simulink model "TempControl_ClosedLoop"  (R2025b)
settings: Solver=FixedStepAuto  StartTime=0.0  StopTime=1000  FixedStep=10e-3  RelTol=1e-3  EnableMultiTasking=on
libraries: mbedblockslib x2
settings Model: ExtModeTrigDuration=10  Creator=Lukas  LastModifiedBy=matte
settings OptimizationCC: EnhancedBackFolding=on  PassReuseOutputArgsAs=Individual arguments  ZeroExternalMemoryAtStartup=off  ZeroInternalMemoryAtStartup=off  MaxStackSize=64  OptimizeBlockOrder=speed  DifferentSizesBufferReuse=on  OptimizationCustomize=off  EfficientTunableParamExpr=on
settings DebuggingCC: ParameterTunabilityLossMsg=error
settings HardwareCC: ProdBitPerPointer=32.0  ProdBitPerSizeT=32.0  ProdBitPerPtrDiffT=32.0  ProdLargestAtomicInteger=Long  ProdLargestAtomicFloat=Double  ProdWordSize=32.0  ProdLongLongMode=on  ProdHWDeviceType=ARM Compatible->ARM Cortex
settings SFSimCC: MATLABDynamicMemAlloc=off
settings RTWCC: SystemTargetFile=ert.tlc  HardwareBoard=STM32 Nucleo F401RE  TemplateMakefile=ert_default_tmf  Toolchain=GNU Tools for ARM Embedded Processors  GPUComputeCapability=3.5  Description=Embedded Coder
settings CodeAppCC: ForceParamTrailComments=on  IgnoreCustomStorageClasses=off  OperatorAnnotations=on  SimulinkDataObjDesc=on  SFDataObjDesc=on  InsertBlockDesc=on
settings ERTTargetCC: ExtModeTransport=3.0  ExtModeStaticAlloc=on  ExtModeStaticAllocSize=2000.0  ExtModeMexFile=ext_xcp  ExtModeIntrfLevel=Level2 - Open  InlinedParameterPlacement=Hierarchical  DynamicArrayContainerType=coder::array  CodeReplacementLibrary=ARM Cortex-M  SupportContinuousTime=on

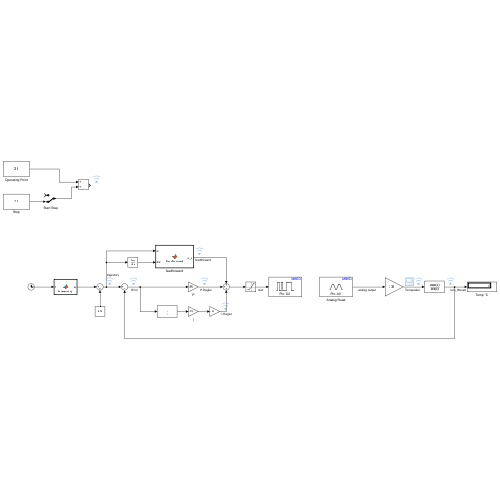
[thumbnail: Simulink's stored preview of the top-level diagram]
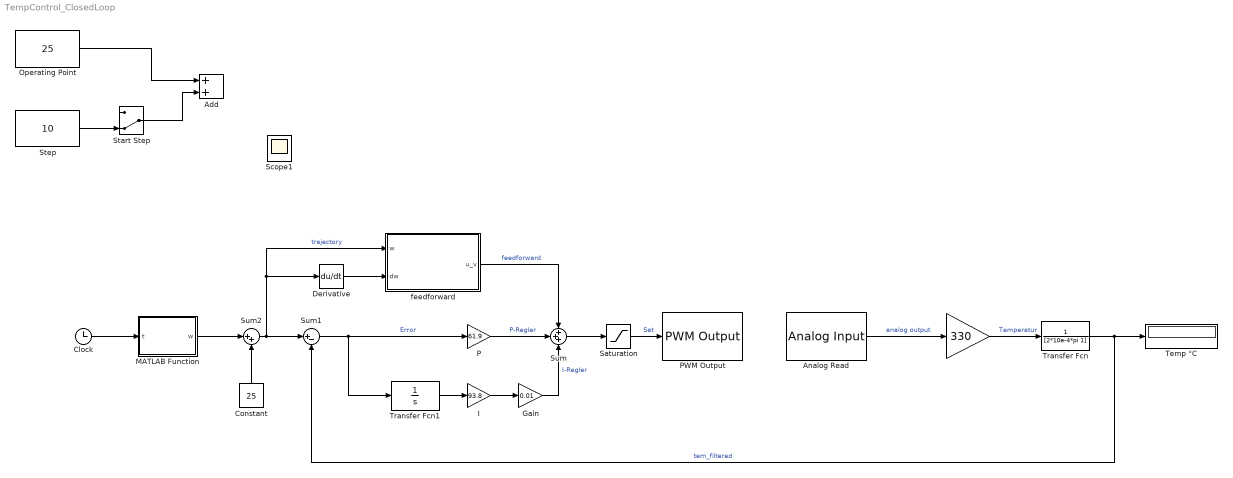
== system TempControl_ClosedLoop ==
  " " : Gain  Gain=330
  Add : Sum
  Analog Read : mbedblockslib/Analog Input  Pin=A0  ReadResultsOnly=off  ConversionTriggerSource=Software  ExternalTriggerType=uint32( 0 )  OutputDataType=double  EnableConversionCompleteNotify=off  EnableOuputStatus=off  SampleTime=10e-3
      settings: LibrarySourceBlock=stmnucleorootlib/Common/Analog Input
  Clock : Clock
  Constant : Constant  Value=25
  Derivative : Derivative
  Gain : Gain  Gain=0.01
  I : Gain  Gain=93.8
  MATLAB Function : MATLAB Function  TreatAsAtomicUnit=on
  Operating Point : Constant  Value=25  SampleTime=10e-3
  P : Gain  Gain=61.9
  PWM Output : mbedblockslib/PWM Output  Pin=D2  EnableInputFrequency=off  InitialFrequency=10000  InitialDutyCycle=20  NotificationType=None
      settings: LibrarySourceBlock=stmnucleorootlib/Common/PWM Output
  Saturation : Saturate  UpperLimit=100  LowerLimit=0
  Start Step : ManualSwitch  CurrentSetting=0
  Step : Constant  Value=10  SampleTime=10e-3
  Sum : Sum  Inputs=+++
  Sum1 : Sum  Inputs=|+-
  Sum2 : Sum  Inputs=|++
  Temp °C : Display
  Transfer Fcn : TransferFcn  Denominator=[2*10e-4*pi 1]
  Transfer Fcn1 : TransferFcn  Denominator=[1 0]
  feedforward : MATLAB Function  TreatAsAtomicUnit=on
  Scope1 : Scope
      settings: ActiveDisplayYMinimum=-1  ActiveDisplayYMaximum=1
  wires:
  Operating Point/1 -> Add/1
  Step/1 -> Start Step/2
  Start Step/1 -> Add/2
  Analog Read/1 -> " "/1  "analog output"
  Saturation/1 -> PWM Output/1  "Sat"
  Sum/1 -> Saturation/1
  Transfer Fcn1/1 -> I/1
  Sum1/1 -> P/1, Transfer Fcn1/1  "Error"
  I/1 -> Gain/1
  MATLAB Function/1(w) -> Sum2/1
  Clock/1 -> MATLAB Function/1(t)
  Derivative/1 -> feedforward/2(dw)
  Gain/1 -> Sum/3  "I-Regler"
  P/1 -> Sum/2  "P-Regler"
  Sum2/1 -> Sum1/1, feedforward/1(w), Derivative/1  "trajectory"
  Constant/1 -> Sum2/2
  feedforward/1(u_v) -> Sum/1  "feedforward"
  " "/1 -> Transfer Fcn/1  "Temperatur"
  Transfer Fcn/1 -> Sum1/2, Temp °C/1  "tem_filtered"

== matlab function TempControl_ClosedLoop/MATLAB Function ==
  data: t input; w output
function w = trajectory(t)
    if t < 80
        w = 15/80 *t;
    elseif t < 120
        w = 15;
    elseif t < 240
        w = -15/120 * (t - 120) + 15;
    else
        w = 0;
    end
end

== matlab function TempControl_ClosedLoop/feedforward ==
  data: w input; u_v output; dw input
function u_v = feedforward(w, dw)

    K = 0.5849;
    T = 130.3;

    u_v = ( T * dw + w) / K;
    
end
